simulink model "Deployed_On_CPU2"  (R2020a)
settings: Solver=ode4  StartTime=0.0  StopTime=Inf  FixedStep=0.01  RelTol=1e-3  EnableMultiTasking=on
undefined symbols (not defined in the file): C28x, CPU1, CPU2
libraries: c280xlib x47, dspobslib x27, simulink x20, c2837xDlib x1
(part 2 of 3)

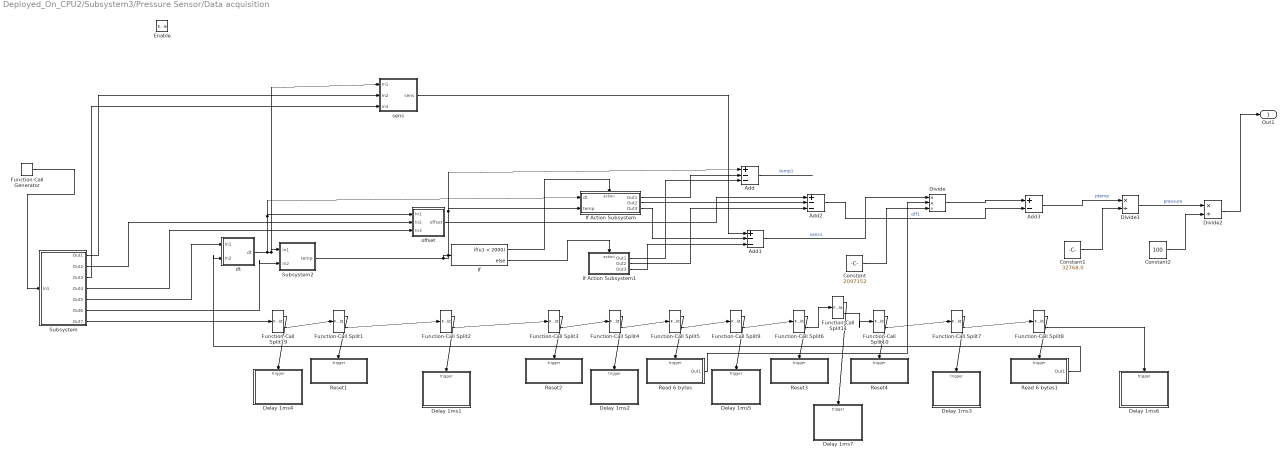
== system Deployed_On_CPU2/Subsystem3/Pressure Sensor/Data acquisition ==
  Enable : EnablePort
  Add : Sum  Inputs=+--
  Add1 : Sum  Inputs=+--
  Add2 : Sum  Inputs=+--
  Add3 : Sum  Inputs=+-
  Constant : Constant  Value=2097152
  Constant1 : Constant  Value=32768.0
  Constant2 : Constant  Value=100
  Delay 1ms1 : Subsystem  TreatAsAtomicUnit=on
  Delay 1ms2 : Subsystem  TreatAsAtomicUnit=on
  Delay 1ms3 : Subsystem  TreatAsAtomicUnit=on
  Delay 1ms4 : Subsystem  TreatAsAtomicUnit=on
  Delay 1ms5 : Subsystem  TreatAsAtomicUnit=on
  Delay 1ms6 : Subsystem  TreatAsAtomicUnit=on
  Delay 1ms7 : Subsystem  TreatAsAtomicUnit=on
  Divide : Product  Inputs=**/
  Divide1 : Product  Inputs=*/
  Divide2 : Product  Inputs=*/
  Function-Call Generator : simulink/Ports & Subsystems/Function-Call Generator  sample_time=0.01  numberOfIterations=1
  Function-Call Split{1..11,19} (12 alike) : FunctionCallSplit  NumOutputPorts=2
  If : If  IfExpression=u1 < 2000
  If Action Subsystem : Subsystem  TreatAsAtomicUnit=on
  If Action Subsystem1 : Subsystem  TreatAsAtomicUnit=on
  Read 6 bytes : Subsystem  TreatAsAtomicUnit=on
  Read 6 bytes1 : Subsystem  TreatAsAtomicUnit=on
  Reset1 : Subsystem  TreatAsAtomicUnit=on
  Reset2 : Subsystem  TreatAsAtomicUnit=on
  Reset3 : Subsystem  TreatAsAtomicUnit=on
  Reset4 : Subsystem  TreatAsAtomicUnit=on
  Subsystem : Subsystem
  Subsystem2 : Subsystem
  dt : Subsystem
  offset : Subsystem
  sens : Subsystem
  Out1 : Outport
  wires:
  Function-Call Split19/1 -> Delay 1ms4/Trigger
  Function-Call Split1/1 -> Reset1/Trigger
  Function-Call Split19/2 -> Function-Call Split1/1
  Function-Call Split2/1 -> Delay 1ms1/Trigger
  Function-Call Split1/2 -> Function-Call Split2/1
  Function-Call Split3/1 -> Reset2/Trigger
  Function-Call Split2/2 -> Function-Call Split3/1
  Function-Call Split4/2 -> Function-Call Split5/1
  Function-Call Split3/2 -> Function-Call Split4/1
  Function-Call Split4/1 -> Delay 1ms2/Trigger
  Function-Call Split5/1 -> Read 6 bytes/Trigger
  Function-Call Split8/1 -> Read 6 bytes1/Trigger
  Function-Call Split7/1 -> Delay 1ms3/Trigger
  Function-Call Split7/2 -> Function-Call Split8/1
  Function-Call Split6/1 -> Reset3/Trigger
  Function-Call Split9/1 -> Delay 1ms5/Trigger
  Function-Call Split5/2 -> Function-Call Split9/1
  Function-Call Split9/2 -> Function-Call Split6/1
  Function-Call Split8/2 -> Delay 1ms6/Trigger
  Function-Call Generator/1 -> Subsystem/1(In1)
  Subsystem/7(Out7) -> Function-Call Split19/1
  Function-Call Split10/1 -> Reset4/Trigger
  Function-Call Split10/2 -> Function-Call Split7/1
  Function-Call Split6/2 -> Function-Call Split11/1
  Function-Call Split11/2 -> Function-Call Split10/1
  Function-Call Split11/1 -> Delay 1ms7/Trigger
  Read 6 bytes1/1(Out1) -> dt/2(In2)
  Subsystem/6(Out6) -> Subsystem2/2(In2)
  Subsystem/2(Out2) -> offset/2(In2)
  Subsystem/4(Out4) -> offset/3(In3)
  dt/1(dt) -> offset/1(In1), If Action Subsystem/1(dt), sens/1(In1), Subsystem2/1(In1)
  Subsystem/5(Out5) -> dt/1(In1)
  Subsystem/1(Out1) -> sens/2(In2)
  Subsystem/3(Out3) -> sens/3(In3)
  Subsystem2/1(temp) -> If Action Subsystem/2(temp), Add/1, If/1
  If/1 -> If Action Subsystem/Action
  If/2 -> If Action Subsystem1/Action
  If Action Subsystem/1(Out1) -> Add/2
  If Action Subsystem1/1(Out1) -> Add/3
  Add/1 -> ?  "temp1"
  offset/1(offset) -> Add2/1
  If Action Subsystem/2(Out2) -> Add2/2
  If Action Subsystem1/2(Out2) -> Add2/3
  sens/1(sens) -> Add1/1
  If Action Subsystem/3(Out3) -> Add1/2
  If Action Subsystem1/3(Out3) -> Add1/3
  Add1/1 -> Divide/1  "sens1"
  Add2/1 -> Add3/2  "off1"
  Read 6 bytes/1(Out1) -> Divide/2
  Constant/1 -> Divide/3
  Divide/1 -> Add3/1
  Add3/1 -> Divide1/1  "ptemp"
  Constant1/1 -> Divide1/2
  Divide1/1 -> Divide2/1  "pressure"
  Constant2/1 -> Divide2/2
  Divide2/1 -> Out1/1

== system Deployed_On_CPU2/Subsystem3/Pressure Sensor/Setup ==
  Enable : EnablePort
  Function-Call Generator : simulink/Ports & Subsystems/Function-Call Generator  sample_time=0.01  numberOfIterations=1
  Function-Call Split : FunctionCallSplit  NumOutputPorts=2
  Reset : Subsystem  TreatAsAtomicUnit=on
  wires:
  Function-Call Split/1 -> Reset/Trigger
  Function-Call Generator/1 -> Function-Call Split/1

== system Deployed_On_CPU2/Subsystem3/Setup/BW_RATE1 ==
  function : TriggerPort  TriggerType=function-call  VariantControl=Variant
  Data : dspobslib/DSP Constant  Value=hex2dec('0A')  SampleMode=Discrete  discreteOutput=Sample-based  continuousOutput=Sample-based  sampTime=-1  framePeriod=2  dataType=uint8  isSigned=on  wordLen=16  udDataType=sfix(16)  fracBitsMode=Best precision  numFracBits=15  InterpretAs1D=-inf  Ts=-inf  FramebasedOutput=-inf
      settings: SourceProductBaseCode=DS
  I2C Transmit : c280xlib/I2C Transmit  selectModule=I2C_A  addrFormat=7-Bit addressing  saSource=Specify via dialog  SAR=83  bitCount=8  STP=on  RM=off  STR=on
      settings: SourceProductBaseCode=TIC2000
  Mux : Mux  Inputs=2
  Register address : dspobslib/DSP Constant  Priority=10  Value=hex2dec('2C')  SampleMode=Discrete  discreteOutput=Sample-based  continuousOutput=Sample-based  sampTime=-1  framePeriod=2  dataType=uint8  isSigned=on  wordLen=16  udDataType=sfix(16)  fracBitsMode=Best precision  numFracBits=15  InterpretAs1D=-inf  Ts=-inf  FramebasedOutput=-inf
      settings: SourceProductBaseCode=DS
  Terminator : Terminator
  wires:
  Mux/1 -> I2C Transmit/1
  I2C Transmit/1 -> Terminator/1
  Register address/1 -> Mux/1
  Data/1 -> Mux/2

== system Deployed_On_CPU2/Subsystem3/Setup/BW_RATE2 ==
  function : TriggerPort  TriggerType=function-call  VariantControl=Variant
  Data : dspobslib/DSP Constant  Value=hex2dec('70')  SampleMode=Discrete  discreteOutput=Sample-based  continuousOutput=Sample-based  sampTime=-1  framePeriod=2  dataType=uint8  isSigned=on  wordLen=16  udDataType=sfix(16)  fracBitsMode=Best precision  numFracBits=15  InterpretAs1D=-inf  Ts=-inf  FramebasedOutput=-inf
      settings: SourceProductBaseCode=DS
  I2C Transmit : c280xlib/I2C Transmit  selectModule=I2C_A  addrFormat=7-Bit addressing  saSource=Specify via dialog  SAR=hex2dec('1E')  bitCount=8  STP=on  RM=off  STR=on
      settings: SourceProductBaseCode=TIC2000
  Mux : Mux  Inputs=2
  Register address : dspobslib/DSP Constant  Priority=10  Value=hex2dec('00')  SampleMode=Discrete  discreteOutput=Sample-based  continuousOutput=Sample-based  sampTime=-1  framePeriod=2  dataType=uint8  isSigned=on  wordLen=16  udDataType=sfix(16)  fracBitsMode=Best precision  numFracBits=15  InterpretAs1D=-inf  Ts=-inf  FramebasedOutput=-inf
      settings: SourceProductBaseCode=DS
  Terminator : Terminator
  wires:
  Mux/1 -> I2C Transmit/1
  I2C Transmit/1 -> Terminator/1
  Register address/1 -> Mux/1
  Data/1 -> Mux/2

== system Deployed_On_CPU2/Subsystem3/Setup/CTRL_REG1 ==
  function : TriggerPort  TriggerType=function-call  VariantControl=Variant
  Data1 : dspobslib/DSP Constant  Value=hex2dec('0A')  SampleMode=Discrete  discreteOutput=Sample-based  continuousOutput=Sample-based  sampTime=-1  framePeriod=2  dataType=uint8  isSigned=on  wordLen=16  udDataType=sfix(16)  fracBitsMode=Best precision  numFracBits=15  InterpretAs1D=-inf  Ts=-inf  FramebasedOutput=-inf
      settings: SourceProductBaseCode=DS
  I2C Transmit : c280xlib/I2C Transmit  selectModule=I2C_A  addrFormat=7-Bit addressing  saSource=Specify via dialog  SAR=hex2dec('69')  bitCount=8  STP=on  RM=off  STR=on
      settings: SourceProductBaseCode=TIC2000
  Mux : Mux  Inputs=2
  Register address : dspobslib/DSP Constant  Priority=10  Value=hex2dec('20')  SampleMode=Discrete  discreteOutput=Sample-based  continuousOutput=Sample-based  sampTime=-1  framePeriod=2  dataType=uint8  isSigned=on  wordLen=16  udDataType=sfix(16)  fracBitsMode=Best precision  numFracBits=15  InterpretAs1D=-inf  Ts=-inf  FramebasedOutput=-inf
      settings: SourceProductBaseCode=DS
  Terminator : Terminator
  wires:
  Register address/1 -> Mux/1
  Mux/1 -> I2C Transmit/1
  Data1/1 -> Mux/2
  I2C Transmit/1 -> Terminator/1

== system Deployed_On_CPU2/Subsystem3/Setup/CTRL_REG2 ==
  function : TriggerPort  TriggerType=function-call  VariantControl=Variant
  Data : dspobslib/DSP Constant  Value=hex2dec('50')  SampleMode=Discrete  discreteOutput=Sample-based  continuousOutput=Sample-based  sampTime=-1  framePeriod=2  dataType=uint8  isSigned=on  wordLen=16  udDataType=sfix(16)  fracBitsMode=Best precision  numFracBits=15  InterpretAs1D=-inf  Ts=-inf  FramebasedOutput=-inf
      settings: SourceProductBaseCode=DS
  I2C Transmit : c280xlib/I2C Transmit  selectModule=I2C_A  addrFormat=7-Bit addressing  saSource=Specify via dialog  SAR=hex2dec('69')  bitCount=8  STP=on  RM=off  STR=on
      settings: SourceProductBaseCode=TIC2000
  Mux : Mux  Inputs=2
  Register address : dspobslib/DSP Constant  Priority=10  Value=hex2dec('24')  SampleMode=Discrete  discreteOutput=Sample-based  continuousOutput=Sample-based  sampTime=-1  framePeriod=2  dataType=uint8  isSigned=on  wordLen=16  udDataType=sfix(16)  fracBitsMode=Best precision  numFracBits=15  InterpretAs1D=-inf  Ts=-inf  FramebasedOutput=-inf
      settings: SourceProductBaseCode=DS
  Terminator : Terminator
  wires:
  Mux/1 -> I2C Transmit/1
  I2C Transmit/1 -> Terminator/1
  Data/1 -> Mux/2
  Register address/1 -> Mux/1

== system Deployed_On_CPU2/Subsystem3/Setup/CTRL_REG4 ==
  note: 250dps
  function : TriggerPort  TriggerType=function-call  VariantControl=Variant
  Data1 : dspobslib/DSP Constant  Value=hex2dec('00')  SampleMode=Discrete  discreteOutput=Sample-based  continuousOutput=Sample-based  sampTime=-1  framePeriod=2  dataType=uint8  isSigned=on  wordLen=16  udDataType=sfix(16)  fracBitsMode=Best precision  numFracBits=15  InterpretAs1D=-inf  Ts=-inf  FramebasedOutput=-inf
      settings: SourceProductBaseCode=DS
  I2C Transmit : c280xlib/I2C Transmit  selectModule=I2C_A  addrFormat=7-Bit addressing  saSource=Specify via dialog  SAR=hex2dec('69')  bitCount=8  STP=on  RM=off  STR=on
      settings: SourceProductBaseCode=TIC2000
  Mux : Mux  Inputs=2
  Register address : dspobslib/DSP Constant  Priority=10  Value=hex2dec('23')  SampleMode=Discrete  discreteOutput=Sample-based  continuousOutput=Sample-based  sampTime=-1  framePeriod=2  dataType=uint8  isSigned=on  wordLen=16  udDataType=sfix(16)  fracBitsMode=Best precision  numFracBits=15  InterpretAs1D=-inf  Ts=-inf  FramebasedOutput=-inf
      settings: SourceProductBaseCode=DS
  Terminator : Terminator
  wires:
  Mux/1 -> I2C Transmit/1
  I2C Transmit/1 -> Terminator/1
  Data1/1 -> Mux/2
  Register address/1 -> Mux/1

== system Deployed_On_CPU2/Subsystem3/Setup/DATA_FORMAT1 ==
  function : TriggerPort  TriggerType=function-call  VariantControl=Variant
  Data : dspobslib/DSP Constant  Value=hex2dec('08')  SampleMode=Discrete  discreteOutput=Sample-based  continuousOutput=Sample-based  sampTime=-1  framePeriod=2  dataType=uint8  isSigned=on  wordLen=16  udDataType=sfix(16)  fracBitsMode=Best precision  numFracBits=15  InterpretAs1D=-inf  Ts=-inf  FramebasedOutput=-inf
      settings: SourceProductBaseCode=DS
  I2C Transmit : c280xlib/I2C Transmit  selectModule=I2C_A  addrFormat=7-Bit addressing  saSource=Specify via dialog  SAR=83  bitCount=8  STP=on  RM=off  STR=on
      settings: SourceProductBaseCode=TIC2000
  Mux : Mux  Inputs=2
  Register address : dspobslib/DSP Constant  Priority=10  Value=hex2dec('31')  SampleMode=Discrete  discreteOutput=Sample-based  continuousOutput=Sample-based  sampTime=-1  framePeriod=2  dataType=uint8  isSigned=on  wordLen=16  udDataType=sfix(16)  fracBitsMode=Best precision  numFracBits=15  InterpretAs1D=-inf  Ts=-inf  FramebasedOutput=-inf
      settings: SourceProductBaseCode=DS
  Terminator : Terminator
  wires:
  Register address/1 -> Mux/1
  Data/1 -> Mux/2
  Mux/1 -> I2C Transmit/1
  I2C Transmit/1 -> Terminator/1

== system Deployed_On_CPU2/Subsystem3/Setup/DATA_FORMAT2 ==
  function : TriggerPort  TriggerType=function-call  VariantControl=Variant
  Data : dspobslib/DSP Constant  Value=hex2dec('00')  SampleMode=Discrete  discreteOutput=Sample-based  continuousOutput=Sample-based  sampTime=-1  framePeriod=2  dataType=uint8  isSigned=on  wordLen=16  udDataType=sfix(16)  fracBitsMode=Best precision  numFracBits=15  InterpretAs1D=-inf  Ts=-inf  FramebasedOutput=-inf
      settings: SourceProductBaseCode=DS
  I2C Transmit : c280xlib/I2C Transmit  selectModule=I2C_A  addrFormat=7-Bit addressing  saSource=Specify via dialog  SAR=hex2dec('1E')  bitCount=8  STP=on  RM=off  STR=on
      settings: SourceProductBaseCode=TIC2000
  Mux : Mux  Inputs=2
  Register address : dspobslib/DSP Constant  Priority=10  Value=hex2dec('02')  SampleMode=Discrete  discreteOutput=Sample-based  continuousOutput=Sample-based  sampTime=-1  framePeriod=2  dataType=uint8  isSigned=on  wordLen=16  udDataType=sfix(16)  fracBitsMode=Best precision  numFracBits=15  InterpretAs1D=-inf  Ts=-inf  FramebasedOutput=-inf
      settings: SourceProductBaseCode=DS
  Terminator : Terminator
  wires:
  Register address/1 -> Mux/1
  Data/1 -> Mux/2
  Mux/1 -> I2C Transmit/1
  I2C Transmit/1 -> Terminator/1

== system Deployed_On_CPU2/Subsystem3/Setup/Delay 1ms10 ==
  function : TriggerPort  TriggerType=function-call  VariantControl=Variant
  System Outputs : Subsystem  mask(System Outputs){ShowInLibBrowser=0}
      mask prompts: ShowInLibBrowser "Simulink:masks:CustCodeMaskParam1_MP"
      settings: CopyFcn=cccopyfcn(gcb)  OpenFcn=ccopenfcn('System Outputs Function')
      mask Help: eval('feval(''rtwprivate'',''rtwhelpview'',''rtw_sys_outputs_block'')');
      mask Display: disp('System\nOutputs');

== system Deployed_On_CPU2/Subsystem3/Setup/Delay 1ms11 ==
  function : TriggerPort  TriggerType=function-call  VariantControl=Variant
  System Outputs : Subsystem  mask(System Outputs){ShowInLibBrowser=0}
      mask prompts: ShowInLibBrowser "Simulink:masks:CustCodeMaskParam1_MP"
      settings: CopyFcn=cccopyfcn(gcb)  OpenFcn=ccopenfcn('System Outputs Function')
      mask Help: eval('feval(''rtwprivate'',''rtwhelpview'',''rtw_sys_outputs_block'')');
      mask Display: disp('System\nOutputs');

== system Deployed_On_CPU2/Subsystem3/Setup/Delay 1ms12 ==
  function : TriggerPort  TriggerType=function-call  VariantControl=Variant
  System Outputs : Subsystem  mask(System Outputs){ShowInLibBrowser=0}
      mask prompts: ShowInLibBrowser "Simulink:masks:CustCodeMaskParam1_MP"
      settings: CopyFcn=cccopyfcn(gcb)  OpenFcn=ccopenfcn('System Outputs Function')
      mask Help: eval('feval(''rtwprivate'',''rtwhelpview'',''rtw_sys_outputs_block'')');
      mask Display: disp('System\nOutputs');

== system Deployed_On_CPU2/Subsystem3/Setup/Delay 1ms13 ==
  function : TriggerPort  TriggerType=function-call  VariantControl=Variant
  System Outputs : Subsystem  mask(System Outputs){ShowInLibBrowser=0}
      mask prompts: ShowInLibBrowser "Simulink:masks:CustCodeMaskParam1_MP"
      settings: CopyFcn=cccopyfcn(gcb)  OpenFcn=ccopenfcn('System Outputs Function')
      mask Help: eval('feval(''rtwprivate'',''rtwhelpview'',''rtw_sys_outputs_block'')');
      mask Display: disp('System\nOutputs');

== system Deployed_On_CPU2/Subsystem3/Setup/Delay 1ms14 ==
  function : TriggerPort  TriggerType=function-call  VariantControl=Variant
  System Outputs : Subsystem  mask(System Outputs){ShowInLibBrowser=0}
      mask prompts: ShowInLibBrowser "Simulink:masks:CustCodeMaskParam1_MP"
      settings: CopyFcn=cccopyfcn(gcb)  OpenFcn=ccopenfcn('System Outputs Function')
      mask Help: eval('feval(''rtwprivate'',''rtwhelpview'',''rtw_sys_outputs_block'')');
      mask Display: disp('System\nOutputs');

== system Deployed_On_CPU2/Subsystem3/Setup/Delay 1ms15 ==
  function : TriggerPort  TriggerType=function-call  VariantControl=Variant
  System Outputs : Subsystem  mask(System Outputs){ShowInLibBrowser=0}
      mask prompts: ShowInLibBrowser "Simulink:masks:CustCodeMaskParam1_MP"
      settings: CopyFcn=cccopyfcn(gcb)  OpenFcn=ccopenfcn('System Outputs Function')
      mask Help: eval('feval(''rtwprivate'',''rtwhelpview'',''rtw_sys_outputs_block'')');
      mask Display: disp('System\nOutputs');

== system Deployed_On_CPU2/Subsystem3/Setup/Delay 1ms16 ==
  function : TriggerPort  TriggerType=function-call  VariantControl=Variant
  System Outputs : Subsystem  mask(System Outputs){ShowInLibBrowser=0}
      mask prompts: ShowInLibBrowser "Simulink:masks:CustCodeMaskParam1_MP"
      settings: CopyFcn=cccopyfcn(gcb)  OpenFcn=ccopenfcn('System Outputs Function')
      mask Help: eval('feval(''rtwprivate'',''rtwhelpview'',''rtw_sys_outputs_block'')');
      mask Display: disp('System\nOutputs');

== system Deployed_On_CPU2/Subsystem3/Setup/Delay 1ms5 ==
  function : TriggerPort  TriggerType=function-call  VariantControl=Variant
  System Outputs : Subsystem  mask(System Outputs){ShowInLibBrowser=0}
      mask prompts: ShowInLibBrowser "Simulink:masks:CustCodeMaskParam1_MP"
      settings: CopyFcn=cccopyfcn(gcb)  OpenFcn=ccopenfcn('System Outputs Function')
      mask Help: eval('feval(''rtwprivate'',''rtwhelpview'',''rtw_sys_outputs_block'')');
      mask Display: disp('System\nOutputs');

== system Deployed_On_CPU2/Subsystem3/Setup/Delay 1ms7 ==
  function : TriggerPort  TriggerType=function-call  VariantControl=Variant
  System Outputs : Subsystem  mask(System Outputs){ShowInLibBrowser=0}
      mask prompts: ShowInLibBrowser "Simulink:masks:CustCodeMaskParam1_MP"
      settings: CopyFcn=cccopyfcn(gcb)  OpenFcn=ccopenfcn('System Outputs Function')
      mask Help: eval('feval(''rtwprivate'',''rtwhelpview'',''rtw_sys_outputs_block'')');
      mask Display: disp('System\nOutputs');

== system Deployed_On_CPU2/Subsystem3/Setup/Delay 1ms8 ==
  function : TriggerPort  TriggerType=function-call  VariantControl=Variant
  System Outputs : Subsystem  mask(System Outputs){ShowInLibBrowser=0}
      mask prompts: ShowInLibBrowser "Simulink:masks:CustCodeMaskParam1_MP"
      settings: CopyFcn=cccopyfcn(gcb)  OpenFcn=ccopenfcn('System Outputs Function')
      mask Help: eval('feval(''rtwprivate'',''rtwhelpview'',''rtw_sys_outputs_block'')');
      mask Display: disp('System\nOutputs');

== system Deployed_On_CPU2/Subsystem3/Setup/Delay 1ms9 ==
  function : TriggerPort  TriggerType=function-call  VariantControl=Variant
  System Outputs : Subsystem  mask(System Outputs){ShowInLibBrowser=0}
      mask prompts: ShowInLibBrowser "Simulink:masks:CustCodeMaskParam1_MP"
      settings: CopyFcn=cccopyfcn(gcb)  OpenFcn=ccopenfcn('System Outputs Function')
      mask Help: eval('feval(''rtwprivate'',''rtwhelpview'',''rtw_sys_outputs_block'')');
      mask Display: disp('System\nOutputs');

== system Deployed_On_CPU2/Subsystem3/Setup/POWER_CTL1 ==
  function : TriggerPort  TriggerType=function-call  VariantControl=Variant
  Data : dspobslib/DSP Constant  Value=hex2dec('08')  SampleMode=Discrete  discreteOutput=Sample-based  continuousOutput=Sample-based  sampTime=-1  framePeriod=2  dataType=uint8  isSigned=on  wordLen=16  udDataType=sfix(16)  fracBitsMode=Best precision  numFracBits=15  InterpretAs1D=-inf  Ts=-inf  FramebasedOutput=-inf
      settings: SourceProductBaseCode=DS
  I2C Transmit : c280xlib/I2C Transmit  selectModule=I2C_A  addrFormat=7-Bit addressing  saSource=Specify via dialog  SAR=83  bitCount=8  STP=on  RM=off  STR=on
      settings: SourceProductBaseCode=TIC2000
  Mux : Mux  Inputs=2
  Register address : dspobslib/DSP Constant  Priority=10  Value=hex2dec('2D')  SampleMode=Discrete  discreteOutput=Sample-based  continuousOutput=Sample-based  sampTime=-1  framePeriod=2  dataType=uint8  isSigned=on  wordLen=16  udDataType=sfix(16)  fracBitsMode=Best precision  numFracBits=15  InterpretAs1D=-inf  Ts=-inf  FramebasedOutput=-inf
      settings: SourceProductBaseCode=DS
  Terminator : Terminator
  wires:
  Register address/1 -> Mux/1
  Data/1 -> Mux/2
  Mux/1 -> I2C Transmit/1
  I2C Transmit/1 -> Terminator/1

== system Deployed_On_CPU2/Subsystem3/Setup/POWER_CTL2 ==
  note: ± 1.3 Ga
  function : TriggerPort  TriggerType=function-call  VariantControl=Variant
  Data : dspobslib/DSP Constant  Value=hex2dec('20')  SampleMode=Discrete  discreteOutput=Sample-based  continuousOutput=Sample-based  sampTime=-1  framePeriod=2  dataType=uint8  isSigned=on  wordLen=16  udDataType=sfix(16)  fracBitsMode=Best precision  numFracBits=15  InterpretAs1D=-inf  Ts=-inf  FramebasedOutput=-inf
      settings: SourceProductBaseCode=DS
  I2C Transmit : c280xlib/I2C Transmit  selectModule=I2C_A  addrFormat=7-Bit addressing  saSource=Specify via dialog  SAR=hex2dec('1E')  bitCount=8  STP=on  RM=off  STR=on
      settings: SourceProductBaseCode=TIC2000
  Mux : Mux  Inputs=2
  Register address : dspobslib/DSP Constant  Priority=10  Value=hex2dec('01')  SampleMode=Discrete  discreteOutput=Sample-based  continuousOutput=Sample-based  sampTime=-1  framePeriod=2  dataType=uint8  isSigned=on  wordLen=16  udDataType=sfix(16)  fracBitsMode=Best precision  numFracBits=15  InterpretAs1D=-inf  Ts=-inf  FramebasedOutput=-inf
      settings: SourceProductBaseCode=DS
  Terminator : Terminator
  wires:
  Register address/1 -> Mux/1
  Data/1 -> Mux/2
  Mux/1 -> I2C Transmit/1
  I2C Transmit/1 -> Terminator/1

== system Deployed_On_CPU2/Subsystem3/Setup/Y_OFFSET1 ==
  function : TriggerPort  TriggerType=function-call  VariantControl=Variant
  Data : dspobslib/DSP Constant  Value=1  SampleMode=Discrete  discreteOutput=Sample-based  continuousOutput=Sample-based  sampTime=-1  framePeriod=2  dataType=uint8  isSigned=on  wordLen=16  udDataType=sfix(16)  fracBitsMode=Best precision  numFracBits=15  InterpretAs1D=-inf  Ts=-inf  FramebasedOutput=-inf
      settings: SourceProductBaseCode=DS
  I2C Transmit : c280xlib/I2C Transmit  selectModule=I2C_A  addrFormat=7-Bit addressing  saSource=Specify via dialog  SAR=83  bitCount=8  STP=on  RM=off  STR=on
      settings: SourceProductBaseCode=TIC2000
  Mux : Mux  Inputs=2
  Register address : dspobslib/DSP Constant  Priority=10  Value=hex2dec('1F')  SampleMode=Discrete  discreteOutput=Sample-based  continuousOutput=Sample-based  sampTime=-1  framePeriod=2  dataType=uint8  isSigned=on  wordLen=16  udDataType=sfix(16)  fracBitsMode=Best precision  numFracBits=15  InterpretAs1D=-inf  Ts=-inf  FramebasedOutput=-inf
      settings: SourceProductBaseCode=DS
  Terminator : Terminator
  wires:
  Mux/1 -> I2C Transmit/1
  Register address/1 -> Mux/1
  Data/1 -> Mux/2
  I2C Transmit/1 -> Terminator/1

== system Deployed_On_CPU2/Subsystem3/Setup/Z_OFFSET1 ==
  function : TriggerPort  TriggerType=function-call  VariantControl=Variant
  Data : dspobslib/DSP Constant  Value=3  SampleMode=Discrete  discreteOutput=Sample-based  continuousOutput=Sample-based  sampTime=-1  framePeriod=2  dataType=uint8  isSigned=on  wordLen=16  udDataType=sfix(16)  fracBitsMode=Best precision  numFracBits=15  InterpretAs1D=-inf  Ts=-inf  FramebasedOutput=-inf
      settings: SourceProductBaseCode=DS
  I2C Transmit : c280xlib/I2C Transmit  selectModule=I2C_A  addrFormat=7-Bit addressing  saSource=Specify via dialog  SAR=83  bitCount=8  STP=on  RM=off  STR=on
      settings: SourceProductBaseCode=TIC2000
  Mux : Mux  Inputs=2
  Register address : dspobslib/DSP Constant  Priority=10  Value=hex2dec('20')  SampleMode=Discrete  discreteOutput=Sample-based  continuousOutput=Sample-based  sampTime=-1  framePeriod=2  dataType=uint8  isSigned=on  wordLen=16  udDataType=sfix(16)  fracBitsMode=Best precision  numFracBits=15  InterpretAs1D=-inf  Ts=-inf  FramebasedOutput=-inf
      settings: SourceProductBaseCode=DS
  Terminator : Terminator
  wires:
  I2C Transmit/1 -> Terminator/1
  Data/1 -> Mux/2
  Register address/1 -> Mux/1
  Mux/1 -> I2C Transmit/1

== system Deployed_On_CPU2/Subsystem3/Data acquisition/Delay 1ms/System Outputs ==

== system Deployed_On_CPU2/Subsystem3/Data acquisition/Delay 1ms1/System Outputs ==

== system Deployed_On_CPU2/Subsystem3/Data acquisition/Delay 1ms10/System Outputs ==

== system Deployed_On_CPU2/Subsystem3/Data acquisition/Delay 1ms11/System Outputs ==

== system Deployed_On_CPU2/Subsystem3/Data acquisition/Delay 1ms12/System Outputs ==

== system Deployed_On_CPU2/Subsystem3/Data acquisition/Delay 1ms13/System Outputs ==

== system Deployed_On_CPU2/Subsystem3/Data acquisition/Delay 1ms14/System Outputs ==

== system Deployed_On_CPU2/Subsystem3/Data acquisition/Delay 1ms15/System Outputs ==

== system Deployed_On_CPU2/Subsystem3/Data acquisition/Delay 1ms16/System Outputs ==

== system Deployed_On_CPU2/Subsystem3/Data acquisition/Delay 1ms17/System Outputs ==

== system Deployed_On_CPU2/Subsystem3/Data acquisition/Delay 1ms18/System Outputs ==

== system Deployed_On_CPU2/Subsystem3/Data acquisition/Delay 1ms5/System Outputs ==

== system Deployed_On_CPU2/Subsystem3/Data acquisition/Delay 1ms6/System Outputs ==

== system Deployed_On_CPU2/Subsystem3/Data acquisition/Delay 1ms7/System Outputs ==

== system Deployed_On_CPU2/Subsystem3/Data acquisition/Delay 1ms8/System Outputs ==

== system Deployed_On_CPU2/Subsystem3/Data acquisition/Delay 1ms9/System Outputs ==

== system Deployed_On_CPU2/Subsystem3/Pressure Sensor/Data acquisition/Delay 1ms1 ==
  function : TriggerPort  TriggerType=function-call  VariantControl=Variant
  System Outputs : Subsystem  mask(System Outputs){ShowInLibBrowser=0}
      mask prompts: ShowInLibBrowser "Simulink:masks:CustCodeMaskParam1_MP"
      settings: CopyFcn=cccopyfcn(gcb)  OpenFcn=ccopenfcn('System Outputs Function')
      mask Help: eval('feval(''rtwprivate'',''rtwhelpview'',''rtw_sys_outputs_block'')');
      mask Display: disp('System\nOutputs');

== system Deployed_On_CPU2/Subsystem3/Pressure Sensor/Data acquisition/Delay 1ms2 ==
  function : TriggerPort  TriggerType=function-call  VariantControl=Variant
  System Outputs : Subsystem  mask(System Outputs){ShowInLibBrowser=0}
      mask prompts: ShowInLibBrowser "Simulink:masks:CustCodeMaskParam1_MP"
      settings: CopyFcn=cccopyfcn(gcb)  OpenFcn=ccopenfcn('System Outputs Function')
      mask Help: eval('feval(''rtwprivate'',''rtwhelpview'',''rtw_sys_outputs_block'')');
      mask Display: disp('System\nOutputs');

== system Deployed_On_CPU2/Subsystem3/Pressure Sensor/Data acquisition/Delay 1ms3 ==
  function : TriggerPort  TriggerType=function-call  VariantControl=Variant
  System Outputs : Subsystem  mask(System Outputs){ShowInLibBrowser=0}
      mask prompts: ShowInLibBrowser "Simulink:masks:CustCodeMaskParam1_MP"
      settings: CopyFcn=cccopyfcn(gcb)  OpenFcn=ccopenfcn('System Outputs Function')
      mask Help: eval('feval(''rtwprivate'',''rtwhelpview'',''rtw_sys_outputs_block'')');
      mask Display: disp('System\nOutputs');

== system Deployed_On_CPU2/Subsystem3/Pressure Sensor/Data acquisition/Delay 1ms4 ==
  function : TriggerPort  TriggerType=function-call  VariantControl=Variant
  System Outputs : Subsystem  mask(System Outputs){ShowInLibBrowser=0}
      mask prompts: ShowInLibBrowser "Simulink:masks:CustCodeMaskParam1_MP"
      settings: CopyFcn=cccopyfcn(gcb)  OpenFcn=ccopenfcn('System Outputs Function')
      mask Help: eval('feval(''rtwprivate'',''rtwhelpview'',''rtw_sys_outputs_block'')');
      mask Display: disp('System\nOutputs');

== system Deployed_On_CPU2/Subsystem3/Pressure Sensor/Data acquisition/Delay 1ms5 ==
  function : TriggerPort  TriggerType=function-call  VariantControl=Variant
  System Outputs : Subsystem  mask(System Outputs){ShowInLibBrowser=0}
      mask prompts: ShowInLibBrowser "Simulink:masks:CustCodeMaskParam1_MP"
      settings: CopyFcn=cccopyfcn(gcb)  OpenFcn=ccopenfcn('System Outputs Function')
      mask Help: eval('feval(''rtwprivate'',''rtwhelpview'',''rtw_sys_outputs_block'')');
      mask Display: disp('System\nOutputs');

== system Deployed_On_CPU2/Subsystem3/Pressure Sensor/Data acquisition/Delay 1ms6 ==
  function : TriggerPort  TriggerType=function-call  VariantControl=Variant
  System Outputs : Subsystem  mask(System Outputs){ShowInLibBrowser=0}
      mask prompts: ShowInLibBrowser "Simulink:masks:CustCodeMaskParam1_MP"
      settings: CopyFcn=cccopyfcn(gcb)  OpenFcn=ccopenfcn('System Outputs Function')
      mask Help: eval('feval(''rtwprivate'',''rtwhelpview'',''rtw_sys_outputs_block'')');
      mask Display: disp('System\nOutputs');

== system Deployed_On_CPU2/Subsystem3/Pressure Sensor/Data acquisition/Delay 1ms7 ==
  function : TriggerPort  TriggerType=function-call  VariantControl=Variant
  System Outputs : Subsystem  mask(System Outputs){ShowInLibBrowser=0}
      mask prompts: ShowInLibBrowser "Simulink:masks:CustCodeMaskParam1_MP"
      settings: CopyFcn=cccopyfcn(gcb)  OpenFcn=ccopenfcn('System Outputs Function')
      mask Help: eval('feval(''rtwprivate'',''rtwhelpview'',''rtw_sys_outputs_block'')');
      mask Display: disp('System\nOutputs');

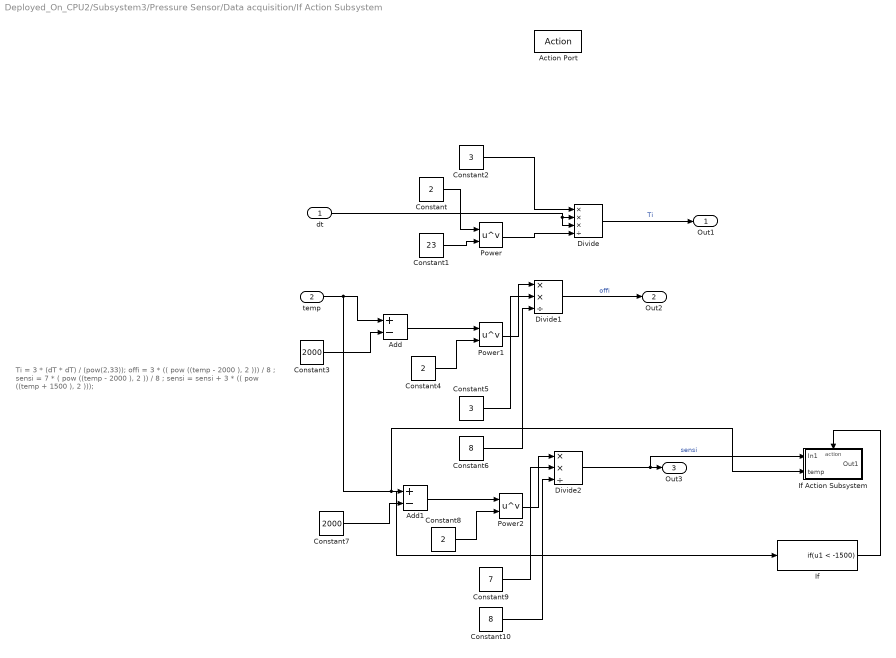
== system Deployed_On_CPU2/Subsystem3/Pressure Sensor/Data acquisition/If Action Subsystem ==
  note: Ti = 3 * (dT * dT) / (pow(2,33));
      | offi = 3 * (( pow ((temp - 2000 ), 2 ))) / 8 ;
      | sensi = 7 * ( pow ((temp - 2000 ), 2 )) / 8 ;
      | sensi = sensi + 3 * (( pow ((temp + 1500 ), 2 )));
  dt : Inport
  temp : Inport  Port=2
  Action Port : ActionPort
  Add : Sum  Inputs=+-
  Add1 : Sum  Inputs=+-
  Constant : Constant  Value=2
  Constant1 : Constant  Value=23
  Constant10 : Constant  Value=8
  Constant2 : Constant  Value=3
  Constant3 : Constant  Value=2000
  Constant4 : Constant  Value=2
  Constant5 : Constant  Value=3
  Constant6 : Constant  Value=8
  Constant7 : Constant  Value=2000
  Constant8 : Constant  Value=2
  Constant9 : Constant  Value=7
  Divide : Product  Inputs=***/
  Divide1 : Product  Inputs=**/
  Divide2 : Product  Inputs=**/
  If : If  IfExpression=u1 < -1500  ShowElse=off
  If Action Subsystem : Subsystem  TreatAsAtomicUnit=on
  Power : Math  Operator=pow  SaturateOnIntegerOverflow=on
  Power1 : Math  Operator=pow  SaturateOnIntegerOverflow=on
  Power2 : Math  Operator=pow  SaturateOnIntegerOverflow=on
  Out1 : Outport
  Out2 : Outport  Port=2
  Out3 : Outport  Port=3
  wires:
  Constant/1 -> Power/1
  Constant1/1 -> Power/2
  Constant2/1 -> Divide/1
  Power/1 -> Divide/4
  dt/1 -> Divide/3, Divide/2
  Divide/1 -> Out1/1  "Ti"
  Constant3/1 -> Add/2
  Add/1 -> Power1/1
  Constant4/1 -> Power1/2
  Power1/1 -> Divide1/1
  Constant5/1 -> Divide1/2
  Constant6/1 -> Divide1/3
  Divide1/1 -> Out2/1  "offi"
  Divide2/1 -> If Action Subsystem/1(In1), Out3/1  "sensi"
  Constant10/1 -> Divide2/3
  Constant9/1 -> Divide2/2
  Power2/1 -> Divide2/1
  Constant8/1 -> Power2/2
  Add1/1 -> Power2/1
  Constant7/1 -> Add1/2
  temp/1 -> If/1, Add1/1, If Action Subsystem/2(temp), Add/1
  If/1 -> If Action Subsystem/Action

== system Deployed_On_CPU2/Subsystem3/Pressure Sensor/Data acquisition/If Action Subsystem1 ==
  Action Port : ActionPort
  Constant : Constant  Value=0
  Constant1 : Constant  Value=0
  Constant2 : Constant  Value=0
  Out1 : Outport
  Out2 : Outport  Port=2
  Out3 : Outport  Port=3
  wires:
  Constant/1 -> Out1/1
  Constant1/1 -> Out2/1
  Constant2/1 -> Out3/1

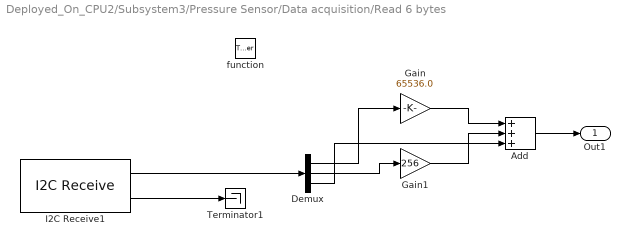
== system Deployed_On_CPU2/Subsystem3/Pressure Sensor/Data acquisition/Read 6 bytes ==
  function : TriggerPort  TriggerType=function-call  VariantControl=Variant
  Add : Sum  Inputs=+++
  Demux : Demux  Outputs=3
  Gain : Gain  Gain=65536.0
  Gain1 : Gain  Gain=256
  I2C Receive1 : c280xlib/I2C Receive  Priority=10  selectModule=I2C_A  addrFormat=7-Bit addressing  saSource=Specify via dialog  SAR=hex2dec('76')  bitCount=8  dataLength=3  initValue=0  NACK=off  STP=on  STR=on  sampleTime=-1  dataType=uint8
      settings: SourceProductBaseCode=TIC2000
  Terminator1 : Terminator
  Out1 : Outport
  wires:
  I2C Receive1/2 -> Terminator1/1
  I2C Receive1/1 -> Demux/1
  Demux/1 -> Gain/1
  Demux/2 -> Gain1/1
  Gain/1 -> Add/1
  Gain1/1 -> Add/2
  Demux/3 -> Add/3
  Add/1 -> Out1/1

== system Deployed_On_CPU2/Subsystem3/Pressure Sensor/Data acquisition/Read 6 bytes1 ==
  function : TriggerPort  TriggerType=function-call  VariantControl=Variant
  Add : Sum  Inputs=+++
  Demux : Demux  Outputs=3
  Gain : Gain  Gain=65536.0
  Gain1 : Gain  Gain=256
  I2C Receive1 : c280xlib/I2C Receive  Priority=10  selectModule=I2C_A  addrFormat=7-Bit addressing  saSource=Specify via dialog  SAR=hex2dec('76')  bitCount=8  dataLength=3  initValue=0  NACK=off  STP=on  STR=on  sampleTime=-1  dataType=uint8
      settings: SourceProductBaseCode=TIC2000
  Terminator1 : Terminator
  Out1 : Outport
  wires:
  Add/1 -> Out1/1
  Demux/3 -> Add/3
  Gain1/1 -> Add/2
  Gain/1 -> Add/1
  Demux/2 -> Gain1/1
  Demux/1 -> Gain/1
  I2C Receive1/1 -> Demux/1
  I2C Receive1/2 -> Terminator1/1

== system Deployed_On_CPU2/Subsystem3/Pressure Sensor/Data acquisition/Reset1 ==
  note: Refresh pressure with the OSR = 256
  function : TriggerPort  TriggerType=function-call  VariantControl=Variant
  Data : dspobslib/DSP Constant  Value=hex2dec('40')  SampleMode=Discrete  discreteOutput=Sample-based  continuousOutput=Sample-based  sampTime=-1  framePeriod=2  dataType=uint8  isSigned=on  wordLen=16  udDataType=sfix(16)  fracBitsMode=Best precision  numFracBits=15  InterpretAs1D=-inf  Ts=-inf  FramebasedOutput=-inf
      settings: SourceProductBaseCode=DS
  I2C Transmit : c280xlib/I2C Transmit  selectModule=I2C_A  addrFormat=7-Bit addressing  saSource=Specify via dialog  SAR=hex2dec('76')  bitCount=8  STP=on  RM=off  STR=on
      settings: SourceProductBaseCode=TIC2000
  Terminator : Terminator
  wires:
  I2C Transmit/1 -> Terminator/1
  Data/1 -> I2C Transmit/1

== system Deployed_On_CPU2/Subsystem3/Pressure Sensor/Data acquisition/Reset2 ==
  note: Refresh pressure with the OSR = 256
  function : TriggerPort  TriggerType=function-call  VariantControl=Variant
  Data : dspobslib/DSP Constant  Value=hex2dec('00')  SampleMode=Discrete  discreteOutput=Sample-based  continuousOutput=Sample-based  sampTime=-1  framePeriod=2  dataType=uint8  isSigned=on  wordLen=16  udDataType=sfix(16)  fracBitsMode=Best precision  numFracBits=15  InterpretAs1D=-inf  Ts=-inf  FramebasedOutput=-inf
      settings: SourceProductBaseCode=DS
  I2C Transmit : c280xlib/I2C Transmit  selectModule=I2C_A  addrFormat=7-Bit addressing  saSource=Specify via dialog  SAR=hex2dec('76')  bitCount=8  STP=on  RM=off  STR=on
      settings: SourceProductBaseCode=TIC2000
  Terminator : Terminator
  wires:
  Data/1 -> I2C Transmit/1
  I2C Transmit/1 -> Terminator/1

== system Deployed_On_CPU2/Subsystem3/Pressure Sensor/Data acquisition/Reset3 ==
  note: Refresh temperature with the OSR = 256
  function : TriggerPort  TriggerType=function-call  VariantControl=Variant
  Data : dspobslib/DSP Constant  Value=hex2dec('50')  SampleMode=Discrete  discreteOutput=Sample-based  continuousOutput=Sample-based  sampTime=-1  framePeriod=2  dataType=uint8  isSigned=on  wordLen=16  udDataType=sfix(16)  fracBitsMode=Best precision  numFracBits=15  InterpretAs1D=-inf  Ts=-inf  FramebasedOutput=-inf
      settings: SourceProductBaseCode=DS
  I2C Transmit : c280xlib/I2C Transmit  selectModule=I2C_A  addrFormat=7-Bit addressing  saSource=Specify via dialog  SAR=hex2dec('76')  bitCount=8  STP=on  RM=off  STR=on
      settings: SourceProductBaseCode=TIC2000
  Terminator : Terminator
  wires:
  I2C Transmit/1 -> Terminator/1
  Data/1 -> I2C Transmit/1

== system Deployed_On_CPU2/Subsystem3/Pressure Sensor/Data acquisition/Reset4 ==
  note: Refresh pressure with the OSR = 256
  function : TriggerPort  TriggerType=function-call  VariantControl=Variant
  Data : dspobslib/DSP Constant  Value=hex2dec('00')  SampleMode=Discrete  discreteOutput=Sample-based  continuousOutput=Sample-based  sampTime=-1  framePeriod=2  dataType=uint8  isSigned=on  wordLen=16  udDataType=sfix(16)  fracBitsMode=Best precision  numFracBits=15  InterpretAs1D=-inf  Ts=-inf  FramebasedOutput=-inf
      settings: SourceProductBaseCode=DS
  I2C Transmit : c280xlib/I2C Transmit  selectModule=I2C_A  addrFormat=7-Bit addressing  saSource=Specify via dialog  SAR=hex2dec('76')  bitCount=8  STP=on  RM=off  STR=on
      settings: SourceProductBaseCode=TIC2000
  Terminator : Terminator
  wires:
  I2C Transmit/1 -> Terminator/1
  Data/1 -> I2C Transmit/1

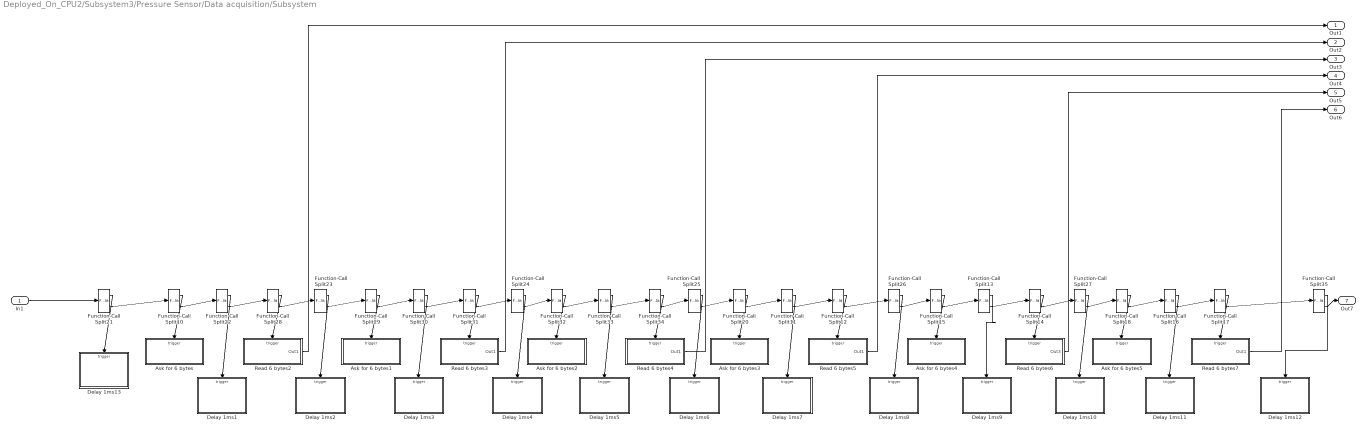
== system Deployed_On_CPU2/Subsystem3/Pressure Sensor/Data acquisition/Subsystem ==
  In1 : Inport
  Ask for 6 bytes : Subsystem  TreatAsAtomicUnit=on
  Ask for 6 bytes1 : Subsystem  TreatAsAtomicUnit=on
  Ask for 6 bytes2 : Subsystem  TreatAsAtomicUnit=on
  Ask for 6 bytes3 : Subsystem  TreatAsAtomicUnit=on
  Ask for 6 bytes4 : Subsystem  TreatAsAtomicUnit=on
  Ask for 6 bytes5 : Subsystem  TreatAsAtomicUnit=on
  Delay 1ms1 : Subsystem  TreatAsAtomicUnit=on
  Delay 1ms10 : Subsystem  TreatAsAtomicUnit=on
  Delay 1ms11 : Subsystem  TreatAsAtomicUnit=on
  Delay 1ms12 : Subsystem  TreatAsAtomicUnit=on
  Delay 1ms13 : Subsystem  TreatAsAtomicUnit=on
  Delay 1ms2 : Subsystem  TreatAsAtomicUnit=on
  Delay 1ms3 : Subsystem  TreatAsAtomicUnit=on
  Delay 1ms4 : Subsystem  TreatAsAtomicUnit=on
  Delay 1ms5 : Subsystem  TreatAsAtomicUnit=on
  Delay 1ms6 : Subsystem  TreatAsAtomicUnit=on
  Delay 1ms7 : Subsystem  TreatAsAtomicUnit=on
  Delay 1ms8 : Subsystem  TreatAsAtomicUnit=on
  Delay 1ms9 : Subsystem  TreatAsAtomicUnit=on
  Function-Call Split{10..18,20..35} (25 alike) : FunctionCallSplit  NumOutputPorts=2
  Read 6 bytes2 : Subsystem  TreatAsAtomicUnit=on
  Read 6 bytes3 : Subsystem  TreatAsAtomicUnit=on
  Read 6 bytes4 : Subsystem  TreatAsAtomicUnit=on
  Read 6 bytes5 : Subsystem  TreatAsAtomicUnit=on
  Read 6 bytes6 : Subsystem  TreatAsAtomicUnit=on
  Read 6 bytes7 : Subsystem  TreatAsAtomicUnit=on
  Out1 : Outport
  Out2 : Outport  Port=2
  Out3 : Outport  Port=3
  Out4 : Outport  Port=4
  Out5 : Outport  Port=5
  Out6 : Outport  Port=6
  Out7 : Outport  Port=7
  wires:
  Read 6 bytes6/1(Out3) -> Out5/1
  Function-Call Split26/1 -> Delay 1ms8/Trigger
  Function-Call Split24/1 -> Delay 1ms4/Trigger
  Function-Call Split33/1 -> Delay 1ms5/Trigger
  Function-Call Split20/2 -> Function-Call Split11/1
  Function-Call Split21/2 -> Function-Call Split10/1
  Function-Call Split35/1 -> Delay 1ms12/Trigger
  Function-Call Split15/1 -> Ask for 6 bytes4/Trigger
  Function-Call Split32/2 -> Function-Call Split33/1
  Function-Call Split14/1 -> Read 6 bytes6/Trigger
  Function-Call Split11/1 -> Delay 1ms7/Trigger
  Function-Call Split34/2 -> Function-Call Split25/1
  Function-Call Split16/2 -> Function-Call Split17/1
  Function-Call Split34/1 -> Read 6 bytes4/Trigger
  Function-Call Split24/2 -> Function-Call Split32/1
  Function-Call Split13/1 -> Delay 1ms9/Trigger
  Function-Call Split28/2 -> Function-Call Split23/1
  Function-Call Split18/1 -> Ask for 6 bytes5/Trigger
  Function-Call Split31/1 -> Read 6 bytes3/Trigger
  Function-Call Split29/2 -> Function-Call Split30/1
  Function-Call Split33/2 -> Function-Call Split34/1
  Function-Call Split32/1 -> Ask for 6 bytes2/Trigger
  Function-Call Split15/2 -> Function-Call Split13/1
  Function-Call Split10/1 -> Ask for 6 bytes/Trigger
  Function-Call Split27/2 -> Function-Call Split18/1
  Function-Call Split30/1 -> Delay 1ms3/Trigger
  Function-Call Split23/2 -> Function-Call Split29/1
  Function-Call Split27/1 -> Delay 1ms10/Trigger
  Function-Call Split31/2 -> Function-Call Split24/1
  Function-Call Split20/1 -> Ask for 6 bytes3/Trigger
  Function-Call Split25/1 -> Delay 1ms6/Trigger
  Function-Call Split18/2 -> Function-Call Split16/1
  Read 6 bytes2/1(Out1) -> Out1/1
  In1/1 -> Function-Call Split21/1
  Function-Call Split29/1 -> Ask for 6 bytes1/Trigger
  Function-Call Split22/1 -> Delay 1ms1/Trigger
  Function-Call Split10/2 -> Function-Call Split22/1
  Function-Call Split17/2 -> Function-Call Split35/1
  Read 6 bytes7/1(Out1) -> Out6/1
  Function-Call Split28/1 -> Read 6 bytes2/Trigger
  Function-Call Split21/1 -> Delay 1ms13/Trigger
  Function-Call Split12/1 -> Read 6 bytes5/Trigger
  Function-Call Split17/1 -> Read 6 bytes7/Trigger
  Function-Call Split30/2 -> Function-Call Split31/1
  Function-Call Split22/2 -> Function-Call Split28/1
  Function-Call Split26/2 -> Function-Call Split15/1
  Function-Call Split12/2 -> Function-Call Split26/1
  Function-Call Split23/1 -> Delay 1ms2/Trigger
  Function-Call Split13/2 -> Function-Call Split14/1
  Function-Call Split14/2 -> Function-Call Split27/1
  Function-Call Split35/2 -> Out7/1
  Function-Call Split25/2 -> Function-Call Split20/1
  Function-Call Split11/2 -> Function-Call Split12/1
  Read 6 bytes4/1(Out1) -> Out3/1
  Function-Call Split16/1 -> Delay 1ms11/Trigger
  Read 6 bytes3/1(Out1) -> Out2/1
  Read 6 bytes5/1(Out1) -> Out4/1

== system Deployed_On_CPU2/Subsystem3/Pressure Sensor/Data acquisition/Subsystem2 ==
  In1 : Inport
  In2 : Inport  Port=2
  Add : Sum
  Constant : Constant  Value=2000
  Divide : Product  Inputs=**/
  Subsystem1 : Subsystem
  temp : Outport
  wires:
  In1/1 -> Divide/1
  Subsystem1/1(Out1) -> Divide/3
  Divide/1 -> Add/2
  Constant/1 -> Add/1
  Add/1 -> temp/1  "temp"
  In2/1 -> Divide/2

== system Deployed_On_CPU2/Subsystem3/Pressure Sensor/Data acquisition/dt ==
  In1 : Inport
  In2 : Inport  Port=2
  Add : Sum  Inputs=+-
  Gain : Gain  Gain=256
  dt : Outport
  wires:
  In1/1 -> Gain/1
  Gain/1 -> Add/2
  In2/1 -> Add/1
  Add/1 -> dt/1  "dt"

== system Deployed_On_CPU2/Subsystem3/Pressure Sensor/Data acquisition/offset ==
  In1 : Inport
  In2 : Inport  Port=2
  In3 : Inport  Port=3
  Add : Sum
  Constant : Constant  Value=32
  Divide : Product  Inputs=**/
  Gain : Gain  Gain=262144
  offset : Outport
  wires:
  In3/1 -> Divide/1
  In2/1 -> Gain/1
  Constant/1 -> Divide/3
  Divide/1 -> Add/2
  Add/1 -> offset/1  "offset"
  In1/1 -> Divide/2
  Gain/1 -> Add/1

== system Deployed_On_CPU2/Subsystem3/Pressure Sensor/Data acquisition/sens ==
  In1 : Inport
  In2 : Inport  Port=2
  In3 : Inport  Port=3
  Add : Sum
  Constant : Constant  Value=128
  Divide : Product  Inputs=**/
  Gain : Gain  Gain=131072
  sens : Outport
  wires:
  In1/1 -> Divide/2
  Divide/1 -> Add/2
  Gain/1 -> Add/1
  Constant/1 -> Divide/3
  Add/1 -> sens/1  "sens"
  In3/1 -> Divide/1
  In2/1 -> Gain/1

== system Deployed_On_CPU2/Subsystem3/Pressure Sensor/Setup/Reset ==
  function : TriggerPort  TriggerType=function-call  VariantControl=Variant
  Data : dspobslib/DSP Constant  Value=hex2dec('1E')  SampleMode=Discrete  discreteOutput=Sample-based  continuousOutput=Sample-based  sampTime=-1  framePeriod=2  dataType=uint8  isSigned=on  wordLen=16  udDataType=sfix(16)  fracBitsMode=Best precision  numFracBits=15  InterpretAs1D=-inf  Ts=-inf  FramebasedOutput=-inf
      settings: SourceProductBaseCode=DS
  I2C Transmit : c280xlib/I2C Transmit  selectModule=I2C_A  addrFormat=7-Bit addressing  saSource=Specify via dialog  SAR=hex2dec('76')  bitCount=8  STP=on  RM=off  STR=on
      settings: SourceProductBaseCode=TIC2000
  Terminator : Terminator
  wires:
  Data/1 -> I2C Transmit/1
  I2C Transmit/1 -> Terminator/1

== system Deployed_On_CPU2/Subsystem3/Setup/Delay 1ms10/System Outputs ==

== system Deployed_On_CPU2/Subsystem3/Setup/Delay 1ms11/System Outputs ==

== system Deployed_On_CPU2/Subsystem3/Setup/Delay 1ms12/System Outputs ==

== system Deployed_On_CPU2/Subsystem3/Setup/Delay 1ms13/System Outputs ==

== system Deployed_On_CPU2/Subsystem3/Setup/Delay 1ms14/System Outputs ==

== system Deployed_On_CPU2/Subsystem3/Setup/Delay 1ms15/System Outputs ==

== system Deployed_On_CPU2/Subsystem3/Setup/Delay 1ms16/System Outputs ==

== system Deployed_On_CPU2/Subsystem3/Setup/Delay 1ms5/System Outputs ==

== system Deployed_On_CPU2/Subsystem3/Setup/Delay 1ms7/System Outputs ==

== system Deployed_On_CPU2/Subsystem3/Setup/Delay 1ms8/System Outputs ==

== system Deployed_On_CPU2/Subsystem3/Setup/Delay 1ms9/System Outputs ==

== system Deployed_On_CPU2/Subsystem3/Pressure Sensor/Data acquisition/Delay 1ms1/System Outputs ==

== system Deployed_On_CPU2/Subsystem3/Pressure Sensor/Data acquisition/Delay 1ms2/System Outputs ==

== system Deployed_On_CPU2/Subsystem3/Pressure Sensor/Data acquisition/Delay 1ms3/System Outputs ==

== system Deployed_On_CPU2/Subsystem3/Pressure Sensor/Data acquisition/Delay 1ms4/System Outputs ==

== system Deployed_On_CPU2/Subsystem3/Pressure Sensor/Data acquisition/Delay 1ms5/System Outputs ==

== system Deployed_On_CPU2/Subsystem3/Pressure Sensor/Data acquisition/Delay 1ms6/System Outputs ==

== system Deployed_On_CPU2/Subsystem3/Pressure Sensor/Data acquisition/Delay 1ms7/System Outputs ==

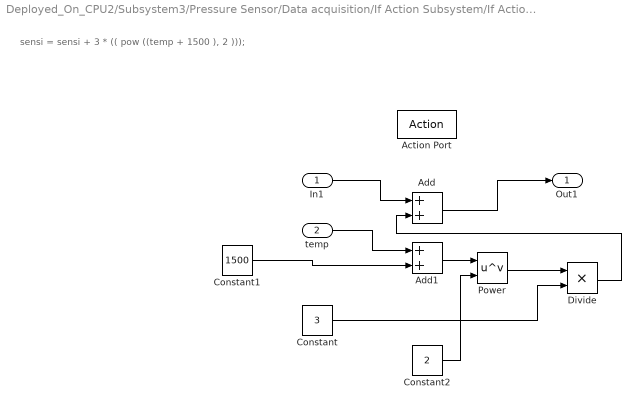
== system Deployed_On_CPU2/Subsystem3/Pressure Sensor/Data acquisition/If Action Subsystem/If Action Subsystem ==
  note: sensi = sensi + 3 * (( pow ((temp + 1500 ), 2 )));
  In1 : Inport
  temp : Inport  Port=2
  Action Port : ActionPort  InitializeStates=reset
  Add : Sum
  Add1 : Sum
  Constant : Constant  Value=3
  Constant1 : Constant  Value=1500
  Constant2 : Constant  Value=2
  Divide : Product  Inputs=**
  Power : Math  Operator=pow  SaturateOnIntegerOverflow=on
  Out1 : Outport
  wires:
  In1/1 -> Add/1
  temp/1 -> Add1/1
  Constant1/1 -> Add1/2
  Add1/1 -> Power/1
  Constant2/1 -> Power/2
  Power/1 -> Divide/1
  Constant/1 -> Divide/2
  Divide/1 -> Add/2
  Add/1 -> Out1/1

== system Deployed_On_CPU2/Subsystem3/Pressure Sensor/Data acquisition/Subsystem/Ask for 6 bytes ==
  function : TriggerPort  TriggerType=function-call  VariantControl=Variant
  Data Read Adress : Constant  Priority=10  Value=hex2dec('A2')  OutDataTypeStr=uint8  SampleTime=-1
  I2C Transmit : c280xlib/I2C Transmit  Priority=20  selectModule=I2C_A  addrFormat=7-Bit addressing  saSource=Specify via dialog  SAR=hex2dec('76')  bitCount=8  STP=on  RM=off  STR=on
      settings: SourceProductBaseCode=TIC2000
  Terminator : Terminator
  wires:
  I2C Transmit/1 -> Terminator/1
  Data Read Adress/1 -> I2C Transmit/1

== system Deployed_On_CPU2/Subsystem3/Pressure Sensor/Data acquisition/Subsystem/Ask for 6 bytes1 ==
  function : TriggerPort  TriggerType=function-call  VariantControl=Variant
  Data Read Adress : Constant  Priority=10  Value=hex2dec('A4')  OutDataTypeStr=uint8  SampleTime=-1
  I2C Transmit : c280xlib/I2C Transmit  Priority=20  selectModule=I2C_A  addrFormat=7-Bit addressing  saSource=Specify via dialog  SAR=hex2dec('76')  bitCount=8  STP=on  RM=off  STR=on
      settings: SourceProductBaseCode=TIC2000
  Terminator : Terminator
  wires:
  Data Read Adress/1 -> I2C Transmit/1
  I2C Transmit/1 -> Terminator/1

== system Deployed_On_CPU2/Subsystem3/Pressure Sensor/Data acquisition/Subsystem/Ask for 6 bytes2 ==
  function : TriggerPort  TriggerType=function-call  VariantControl=Variant
  Data Read Adress : Constant  Priority=10  Value=hex2dec('A6')  OutDataTypeStr=uint8  SampleTime=-1
  I2C Transmit : c280xlib/I2C Transmit  Priority=20  selectModule=I2C_A  addrFormat=7-Bit addressing  saSource=Specify via dialog  SAR=hex2dec('76')  bitCount=8  STP=on  RM=off  STR=on
      settings: SourceProductBaseCode=TIC2000
  Terminator : Terminator
  wires:
  I2C Transmit/1 -> Terminator/1
  Data Read Adress/1 -> I2C Transmit/1

== system Deployed_On_CPU2/Subsystem3/Pressure Sensor/Data acquisition/Subsystem/Ask for 6 bytes3 ==
  function : TriggerPort  TriggerType=function-call  VariantControl=Variant
  Data Read Adress : Constant  Priority=10  Value=hex2dec('A8')  OutDataTypeStr=uint8  SampleTime=-1
  I2C Transmit : c280xlib/I2C Transmit  Priority=20  selectModule=I2C_A  addrFormat=7-Bit addressing  saSource=Specify via dialog  SAR=hex2dec('76')  bitCount=8  STP=on  RM=off  STR=on
      settings: SourceProductBaseCode=TIC2000
  Terminator : Terminator
  wires:
  Data Read Adress/1 -> I2C Transmit/1
  I2C Transmit/1 -> Terminator/1

== system Deployed_On_CPU2/Subsystem3/Pressure Sensor/Data acquisition/Subsystem/Ask for 6 bytes4 ==
  function : TriggerPort  TriggerType=function-call  VariantControl=Variant
  Data Read Adress : Constant  Priority=10  Value=hex2dec('AA')  OutDataTypeStr=uint8  SampleTime=-1
  I2C Transmit : c280xlib/I2C Transmit  Priority=20  selectModule=I2C_A  addrFormat=7-Bit addressing  saSource=Specify via dialog  SAR=hex2dec('76')  bitCount=8  STP=on  RM=off  STR=on
      settings: SourceProductBaseCode=TIC2000
  Terminator : Terminator
  wires:
  I2C Transmit/1 -> Terminator/1
  Data Read Adress/1 -> I2C Transmit/1

== system Deployed_On_CPU2/Subsystem3/Pressure Sensor/Data acquisition/Subsystem/Ask for 6 bytes5 ==
  function : TriggerPort  TriggerType=function-call  VariantControl=Variant
  Data Read Adress : Constant  Priority=10  Value=hex2dec('AC')  OutDataTypeStr=uint8  SampleTime=-1
  I2C Transmit : c280xlib/I2C Transmit  Priority=20  selectModule=I2C_A  addrFormat=7-Bit addressing  saSource=Specify via dialog  SAR=hex2dec('76')  bitCount=8  STP=on  RM=off  STR=on
      settings: SourceProductBaseCode=TIC2000
  Terminator : Terminator
  wires:
  Data Read Adress/1 -> I2C Transmit/1
  I2C Transmit/1 -> Terminator/1

== system Deployed_On_CPU2/Subsystem3/Pressure Sensor/Data acquisition/Subsystem/Delay 1ms1 ==
  function : TriggerPort  TriggerType=function-call  VariantControl=Variant
  System Outputs : Subsystem  mask(System Outputs){ShowInLibBrowser=0}
      mask prompts: ShowInLibBrowser "Simulink:masks:CustCodeMaskParam1_MP"
      settings: CopyFcn=cccopyfcn(gcb)  OpenFcn=ccopenfcn('System Outputs Function')
      mask Help: eval('feval(''rtwprivate'',''rtwhelpview'',''rtw_sys_outputs_block'')');
      mask Display: disp('System\nOutputs');
